simulink model "crazyflie"  (R2015b)
settings: Solver=FixedStepAuto  StartTime=0.0  StopTime=18  FixedStep=1/500  MinStep=1e-4  RelTol=1e-3
undefined symbols (not defined in the file): A, B, C, D
libraries: simulink x1
(part 3 of 3)

== matlab function crazyflie/Off-board ILQR Position Controller/ILQR/MATLAB Function ==
  data: state input; u_new output; setpoint input; u_prev input
function u_new = cf_ilqr(state,setpoint,u_prev)
%#codegen

%% Initialize & Parameters

% CF Parameters
m = 0.041;
g = 9.81;
ct = 3.836E-10;

% ILQR Parameters
N1 = 12; % # of steps
dt = 1/500/12; % time step
Q = diag([0,0,0,0,0,0,0]);
Qf = diag([10000,10000,10000,10000,10000,100,100]);
R = diag([.0001,.0001,.00000001,.0001]);

% Linearized Equtions
A = cell(N1,1);
B = cell(N1,1);

Asym = [1, 0, 0, dt, 0, 0, 0; ...
        0, 1, 0, 0, dt, 0, 0; ...
        0, 0, 1, 0, 0, dt, 0; ...
        0, 0, 0, 1, 0, 0, 0; ...
        0, 0, 0, 0, 1, 0, 0; ...
        0, 0, 0, 0, 0, 1, 0; ...
        0, 0, 0, 0, 0, 0, 1];
    
Bsym = [0, 0, 0, 0; ...
        0, 0, 0, 0; ...
        0, 0, 0, 0; ...
        dt*g, 0, 0, 0; ...
        0, dt*g, 0, 0; ...
        0, 0, (8*dt*sqrt(ct*g*m))/m, 0; ...
        0, 0, 0, dt];
    
for jj = 1:N1
   A{jj} = Asym;
   B{jj} = Bsym;
end

% Initialize ILQR
X = cell(N1+1,1); %state
X{1} = state;
U = cell(N1+1,1); %control effort
U{1} = u_prev;
delta_U = cell(N1+1,1); %change in control effort
delta_U{1} = zeros(4,1);

for jj = 2:N1+1
    X{jj} = zeros(7,1);
    U{jj} = zeros(4,1);
    delta_U{jj} = zeros(4,1);
end

xN = setpoint; %setpoint
S = cell(N1+1,1);
S{N1+1} = Qf;
v = cell(N1+1,1);
K = cell(N1+1,1);
KV = cell(N1+1,1);
KU = cell(N1+1,1);

for jj = 1:N1
   S{jj} = zeros(7,7);
end

for jj = 1:N1+1
   v{jj} = zeros(7,1);
   K{jj} = zeros(4,7);
   KV{jj} = zeros(4,7);
   KU{jj} = zeros(4,4);
end

epsilon = 1E-5;
maxiter = 5;
i = 0;
J_prev = 0;
J_new = 0;

%% Run ILQR

while i < 2 
    %Forward Pass
    for k = 1:N1
       A{k} = Asym;
       B{k} = Bsym;
       X{k+1} = [X{k}(1)+X{k}(4)*dt; ...
                 X{k}(2)+X{k}(5)*dt; ...
                 X{k}(3)+X{k}(6)*dt; ...
                 X{k}(4)+g*dt*U{k}(1); ...
                 X{k}(5)+g*dt*U{k}(2); ...
                 X{k}(6)+8*sqrt(ct*m*g)/m*dt*U{k}(3); ...
                 X{k}(7)+U{k}(4)*dt];
    end
    v{N1+1} = Qf*(X{N1+1} - xN);
    
    % Backward Pass
    for k = N1:-1:1
       K{k} = inv(B{k}'*S{k+1}*B{k}+R)*B{k}'*S{k+1}*A{k};
       KV{k} = inv(B{k}'*S{k+1}*B{k}+R)*B{k}';
       KU{k} = inv(B{k}'*S{k+1}*B{k}+R)*R;
       S{k} = A{k}'*S{k+1}*(A{k}-B{k}*K{k})+Q;
       v{k} = (A{k}-B{k}*K{k})'*v{k+1} - K{k}'*R*U{k} + Q*X{k};
    end
    
    % Update Controls
    for k = 1:N1
       delta_U{k} = (-K{k}*1E-10*ones(7,1) - KV{k}*v{k+1} - KU{k}*U{k});
       U{k} = U{k} + delta_U{k}; 
    end
    
     %Forward Pass
    for k = 1:N1
       A{k} = Asym;
       B{k} = Bsym;
       X{k+1} = [X{k}(1)+X{k}(4)*dt; ...
                 X{k}(2)+X{k}(5)*dt; ...
                 X{k}(3)+X{k}(6)*dt; ...
                 X{k}(4)+g*dt*U{k}(1); ...
                 X{k}(5)+g*dt*U{k}(2); ...
                 X{k}(6)+8*sqrt(ct*m*g)/m*dt*U{k}(3); ...
                 X{k}(7)+U{k}(4)*dt];
    end
    
    % Cost Function
    J_prev = J_new;
    J_new = (X{N1+1} - xN)'*Qf*(X{N1+1} - xN);
    for k = 1:N1+1
       J_new = J_new + U{k}'*R*U{k};
    end
    J_new = .5*J_new;
    
    i = i + 1; % increment
end

while abs(J_prev - J_new) > epsilon && i < maxiter
        %Forward Pass
    for k = 1:N1
       A{k} = Asym;
       B{k} = Bsym;
       X{k+1} = [X{k}(1)+X{k}(4)*dt; ...
                 X{k}(2)+X{k}(5)*dt; ...
                 X{k}(3)+X{k}(6)*dt; ...
                 X{k}(4)+g*dt*U{k}(1); ...
                 X{k}(5)+g*dt*U{k}(2); ...
                 X{k}(6)+8*sqrt(ct*m*g)/m*dt*U{k}(3); ...
                 X{k}(7)+U{k}(4)*dt];
    end
    v{N1+1} = Qf*(X{N1+1} - xN);
    
    % Backward Pass
    for k = N1:-1:1
       K{k} = inv(B{k}'*S{k+1}*B{k}+R)*B{k}'*S{k+1}*A{k};
       KV{k} = inv(B{k}'*S{k+1}*B{k}+R)*B{k}';
       KU{k} = inv(B{k}'*S{k+1}*B{k}+R)*R;
       S{k} = A{k}'*S{k+1}*(A{k}-B{k}*K{k})+Q;
       v{k} = (A{k}-B{k}*K{k})'*v{k+1}-K{k}'*R*U{k}+Q*X{k};
    end
    
    % Update Controls
    for k = 1:N1
       delta_U{k} = (-K{k}*1E-10*ones(7,1) - KV{k}*v{k+1} - KU{k}*U{k});
       U{k} = U{k} + delta_U{k}; 
    end
    
     %Forward Pass
    for k = 1:N1
       A{k} = Asym;
       B{k} = Bsym;
       X{k+1} = [X{k}(1)+X{k}(4)*dt; ...
                 X{k}(2)+X{k}(5)*dt; ...
                 X{k}(3)+X{k}(6)*dt; ...
                 X{k}(4)+g*dt*U{k}(1); ...
                 X{k}(5)+g*dt*U{k}(2); ...
                 X{k}(6)+8*sqrt(ct*m*g)/m*dt*U{k}(3); ...
                 X{k}(7)+U{k}(4)*dt];
    end
    
    % Cost Function
    J_prev = J_new;
    J_new = (X{N1+1} - xN)'*Qf*(X{N1+1} - xN);
    for k = 1:N1+1
       J_new = J_new + U{k}'*R*U{k};
    end
    J_new = .5*J_new;
    
    i = i + 1; % increment
end

u_new = U{1};

== matlab function crazyflie/Off-board LQR Position Controller /Subsystem1/MATLAB Function ==
  data: yaw input; R_m output
function R_m = Error_transform(yaw)
%#codegen

R_m = [cos(yaw) sin(yaw); -sin(yaw) cos(yaw)];

== matlab function crazyflie/Dynamics3/Acceleration ==
  data: F1 input double; F2 input; F3 input; F4 input; r_dot_dot output; rpy input
function r_dot_dot = Crazyflie_accel(F1,F2,F3,F4,rpy)
%#codegen
r_dot_dot = zeros(3,1);
m = 0.041;
g = [0;0;-9.81];

Wrb = [cos(rpy(3))*cos(rpy(2))+sin(rpy(1))*sin(rpy(2))*sin(rpy(3)) -cos(rpy(1))*sin(rpy(3)) cos(rpy(3))*sin(rpy(2))-cos(rpy(2))*sin(rpy(1))*sin(rpy(3)); ...
       cos(rpy(2))*sin(rpy(3))-cos(rpy(3))*sin(rpy(1))*sin(rpy(2)) cos(rpy(1))*cos(rpy(3)) sin(rpy(3))*sin(rpy(2))+cos(rpy(3))*cos(rpy(2))*sin(rpy(1)); ...
       -cos(rpy(1))*sin(rpy(2)) -sin(rpy(1)) cos(rpy(1))*cos(rpy(2))];  
r_dot_dot = g + 1/m * Wrb*[0;0;sum([F1 F2 F3 F4])];

== matlab function crazyflie/Off-board ILQR Position Controller/Subsystem2/MATLAB Function ==
  data: yaw input; R_m output
function R_m = Error_transform(yaw)
%#codegen

R_m = [cos(yaw) sin(yaw); -sin(yaw) cos(yaw)];

== matlab function crazyflie/Dynamics3/Acceleration1 ==
  data: pqr input; rpy_dot output; rpy input
function rpy_dot = Crazyflie_rpy(pqr, rpy)
%#codegen
rpy_dot = zeros(3,1);
Wrb = [cos(rpy(2)) 0 -cos(rpy(1))*sin(rpy(2)); ...
       0 1 sin(rpy(1)); ...
       sin(rpy(2)) 0 cos(rpy(1))*cos(rpy(2))];
  
rpy_dot = Wrb\pqr;

== matlab function crazyflie/Dynamics3/Angular Acceleration ==
  data: F1 input double [0..1]; pqr_dot_x output; F2 input double [0..1]; F3 input double [0..1]; F4 input double [0..1]; M1 input; M2 input; M3 input; M4 input; pqr input
function pqr_dot_x = Crazyflie_ang(F1,F2,F3,F4,M1,M2,M3,M4,pqr)
%#codegen
pqr_dot_x = zeros(3,1);
L = 0.0455;
Ixx = 2.3951E-05;
Iyy = 2.3951E-05;
Izz = 3.2347E-05;
I_matrix = diag([Ixx Iyy Izz]);

Eq1 = [L/sqrt(2)*(F3+F4-F1-F2); ...
      L/sqrt(2)*(F1+F4-F2-F3); ...
      -M1+M2-M3+M4];
Eq2 = cross(pqr, I_matrix*pqr);
  
pqr_dot = inv(I_matrix)*(Eq1 - Eq2);


pqr_dot_x = pqr_dot;

== matlab function crazyflie/Off-board ILQR Position Controller1/ILQR/MATLAB Function ==
  data: state input; u_new output; setpoint input; u_prev input
function u_new = cf_ilqr1(state,setpoint,u_prev)
%#codegen

%% Initialize & Parameters

% CF Parameters
m = 0.041;
g = 9.81;
ct = 3.836E-10;

% ILQR Parameters
N1 = 12; % # of steps
dt = 1/500/12; % time step
Q = diag([0,0,0,0,0,0,0,0,0,0]);
Qf = diag([10000,10000,10000,10000,10000,100,100,10000,10000,100]);
R = diag([.0001,.0001,.00000001,.0001]);

% Linearized Equtions
A = cell(N1,1);
B = cell(N1,1);

Asym = [1, 0, 0, dt, 0, 0, 0, 0, 0, 0; ...
        0, 1, 0, 0, dt, 0, 0, 0, 0, 0; ...
        0, 0, 1, 0, 0, dt, 0, 0, 0, 0; ...
        0, 0, 0, 1, 0, 0, 0, 0, 0, 0; ...
        0, 0, 0, 0, 1, 0, 0, 0, 0, 0,; ...
        0, 0, 0, 0, 0, 1, 0, 0, 0, 0; ...
        0, 0, 0, 0, 0, 0, 1, 0, 0, 0; ...
        0, 0, 0, 0, 0, 0, 0, 1, 0, 0; ...
        0, 0, 0, 0, 0, 0, 0, 0, 1, 0; ...
        0, 0, 0, 0, 0, 0, 0, 0, 0, 1];
    
Bsym = [0, 0, 0, 0; ...
        0, 0, 0, 0; ...
        0, 0, 0, 0; ...
        dt*g, 0, 0, 0; ...
        0, dt*g, 0, 0; ...
        0, 0, (8*dt*sqrt(ct*g*m))/m, 0; ...
        0, 0, 0, dt; ...
        0, 0, 0, 0; ...
        0, 0, 0, 0; ...
        0, 0, 0, 0];
    
for jj = 1:N1
   A{jj} = Asym;
   B{jj} = Bsym;
end

% Initialize ILQR
X = cell(N1+1,1); %state
X{1} = state;
U = cell(N1+1,1); %control effort
U{1} = u_prev;
delta_U = cell(N1+1,1); %change in control effort
delta_U{1} = zeros(4,1);

for jj = 2:N1+1
    X{jj} = zeros(10,1);
    U{jj} = zeros(4,1);
    delta_U{jj} = zeros(4,1);
end

xN = setpoint; %setpoint
S = cell(N1+1,1);
S{N1+1} = Qf;
v = cell(N1+1,1);
K = cell(N1+1,1);
KV = cell(N1+1,1);
KU = cell(N1+1,1);

for jj = 1:N1
   S{jj} = zeros(10,10);
end

for jj = 1:N1+1
   v{jj} = zeros(10,1);
   K{jj} = zeros(4,10);
   KV{jj} = zeros(4,10);
   KU{jj} = zeros(4,4);
end

epsilon = 1E-5;
maxiter = 5;
i = 0;
J_prev = 0;
J_new = 0;

%% Run ILQR

while i < 2 
    %Forward Pass
    for k = 1:N1
       A{k} = Asym;
       B{k} = Bsym;
       X{k+1} = [X{k}(1)+X{k}(4)*dt; ...
                 X{k}(2)+X{k}(5)*dt; ...
                 X{k}(3)+X{k}(6)*dt; ...
                 X{k}(4)+g*dt*U{k}(1); ...
                 X{k}(5)+g*dt*U{k}(2); ...
                 X{k}(6)+8*sqrt(ct*m*g)/m*dt*U{k}(3); ...
                 X{k}(7)+U{k}(4)*dt; ...
                 X{k}(8)-(xN(1)-X{k}(1))*dt; ...
                 X{k}(9)-(xN(2)-X{k}(2))*dt; ...
                 X{k}(10)-(xN(3)-X{k}(3))*dt];
    end
    v{N1+1} = Qf*(X{N1+1} - xN);
    
    % Backward Pass
    for k = N1:-1:1
       K{k} = inv(B{k}'*S{k+1}*B{k}+R)*B{k}'*S{k+1}*A{k};
       KV{k} = inv(B{k}'*S{k+1}*B{k}+R)*B{k}';
       KU{k} = inv(B{k}'*S{k+1}*B{k}+R)*R;
       S{k} = A{k}'*S{k+1}*(A{k}-B{k}*K{k})+Q;
       v{k} = (A{k}-B{k}*K{k})'*v{k+1} - K{k}'*R*U{k} + Q*X{k};
    end
    
    % Update Controls
    for k = 1:N1
       delta_U{k} = (-K{k}*1E-10*ones(10,1) - KV{k}*v{k+1} - KU{k}*U{k});
       U{k} = U{k} + delta_U{k}; 
    end
    
     %Forward Pass
    for k = 1:N1
       A{k} = Asym;
       B{k} = Bsym;
       X{k+1} = [X{k}(1)+X{k}(4)*dt; ...
                 X{k}(2)+X{k}(5)*dt; ...
                 X{k}(3)+X{k}(6)*dt; ...
                 X{k}(4)+g*dt*U{k}(1); ...
                 X{k}(5)+g*dt*U{k}(2); ...
                 X{k}(6)+8*sqrt(ct*m*g)/m*dt*U{k}(3); ...
                 X{k}(7)+U{k}(4)*dt; ...
                 X{k}(8)-(xN(1)-X{k}(1))*dt; ...
                 X{k}(9)-(xN(2)-X{k}(2))*dt; ...
                 X{k}(10)-(xN(3)-X{k}(3))*dt];
    end
    
    % Cost Function
    J_prev = J_new;
    J_new = (X{N1+1} - xN)'*Qf*(X{N1+1} - xN);
    for k = 1:N1+1
       J_new = J_new + U{k}'*R*U{k};
    end
    J_new = .5*J_new;
    
    i = i + 1; % increment
end

while abs(J_prev - J_new) > epsilon && i < maxiter
        %Forward Pass
    for k = 1:N1
       A{k} = Asym;
       B{k} = Bsym;
       X{k+1} = [X{k}(1)+X{k}(4)*dt; ...
                 X{k}(2)+X{k}(5)*dt; ...
                 X{k}(3)+X{k}(6)*dt; ...
                 X{k}(4)+g*dt*U{k}(1); ...
                 X{k}(5)+g*dt*U{k}(2); ...
                 X{k}(6)+8*sqrt(ct*m*g)/m*dt*U{k}(3); ...
                 X{k}(7)+U{k}(4)*dt; ...
                 X{k}(8)-(xN(1)-X{k}(1))*dt; ...
                 X{k}(9)-(xN(2)-X{k}(2))*dt; ...
                 X{k}(10)-(xN(3)-X{k}(3))*dt];
    end
    v{N1+1} = Qf*(X{N1+1} - xN);
    
    % Backward Pass
    for k = N1:-1:1
       K{k} = inv(B{k}'*S{k+1}*B{k}+R)*B{k}'*S{k+1}*A{k};
       KV{k} = inv(B{k}'*S{k+1}*B{k}+R)*B{k}';
       KU{k} = inv(B{k}'*S{k+1}*B{k}+R)*R;
       S{k} = A{k}'*S{k+1}*(A{k}-B{k}*K{k})+Q;
       v{k} = (A{k}-B{k}*K{k})'*v{k+1}-K{k}'*R*U{k}+Q*X{k};
    end
    
    % Update Controls
    for k = 1:N1
       delta_U{k} = (-K{k}*1E-10*ones(10,1) - KV{k}*v{k+1} - KU{k}*U{k});
       U{k} = U{k} + delta_U{k}; 
    end
    
     %Forward Pass
    for k = 1:N1
       A{k} = Asym;
       B{k} = Bsym;
       X{k+1} = [X{k}(1)+X{k}(4)*dt; ...
                 X{k}(2)+X{k}(5)*dt; ...
                 X{k}(3)+X{k}(6)*dt; ...
                 X{k}(4)+g*dt*U{k}(1); ...
                 X{k}(5)+g*dt*U{k}(2); ...
                 X{k}(6)+8*sqrt(ct*m*g)/m*dt*U{k}(3); ...
                 X{k}(7)+U{k}(4)*dt; ...
                 X{k}(8)-(xN(1)-X{k}(1))*dt; ...
                 X{k}(9)-(xN(2)-X{k}(2))*dt; ...
                 X{k}(10)-(xN(3)-X{k}(3))*dt];
    end
    
    % Cost Function
    J_prev = J_new;
    J_new = (X{N1+1} - xN)'*Qf*(X{N1+1} - xN);
    for k = 1:N1+1
       J_new = J_new + U{k}'*R*U{k};
    end
    J_new = .5*J_new;
    
    i = i + 1; % increment
end

u_new = U{1};

== matlab function crazyflie/Off-board ILQR Position Controller1/Subsystem2/MATLAB Function ==
  data: yaw input; R_m output
function R_m = Error_transform(yaw)
%#codegen

R_m = [cos(yaw) sin(yaw); -sin(yaw) cos(yaw)];
